simulink model "exp_9_A"  (R2020b)
settings: Solver=VariableStepAuto  StartTime=0.0  StopTime=10.0  RelTol=1e-3
settings Model: Creator=SWARUP  LastModifiedBy=SWARUP

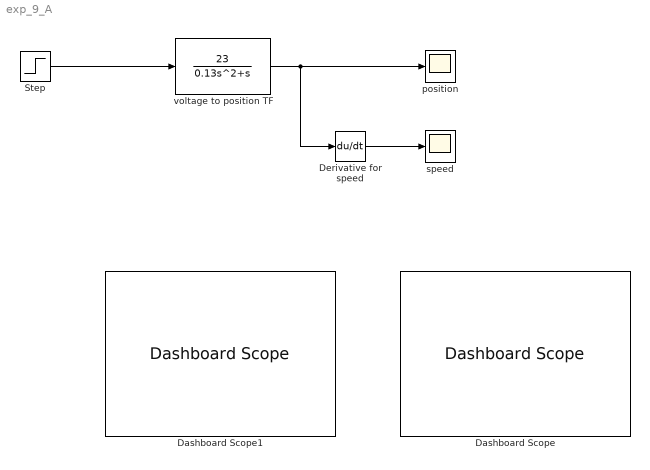
== system exp_9_A ==
  Dashboard Scope : DashboardScope
  Dashboard Scope1 : DashboardScope
  Derivative for speed : Derivative
  Step : Step  SampleTime=0
  position : Scope
  speed : Scope
  voltage to position TF : TransferFcn  Numerator=[23]  Denominator=[0.13 1 0]
  wires:
  voltage to position TF/1 -> Derivative for speed/1, position/1
  Step/1 -> voltage to position TF/1
  Derivative for speed/1 -> speed/1
